simulink model "Gyrometer_model"  (R2015a)
settings: Solver=ode45  StartTime=0.0  StopTime=10.0  RelTol=1e-3
InitFcn:
  | Gyrometer_config;
undefined symbols (not defined in the file or in its folder): gyrometer
libraries: simulink x1
settings Model: Creator=hamada  LastModifiedBy=hamada

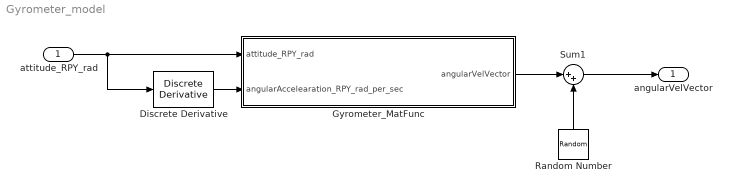
== system Gyrometer_model ==
  attitude_RPY_rad : Inport  PortDimensions=3
  Discrete Derivative : simulink/Discrete/Discrete Derivative  gainval=1.0  ICPrevScaledInput=0.0  InputProcessing=Inherited  OutMin=[]  OutMax=[]  OutDataType=fixdt(1, 16)  OutScaling=2^-10  DoSatur=off
  Gyrometer_MatFunc : MATLAB Function  TreatAsAtomicUnit=on
  Random Number : RandomNumber  Mean=gyrometer.bias  Variance=gyrometer.variance  SampleTime=gyrometer.period
  Sum1 : Sum  Inputs=|++
  angularVelVector : Outport
  wires:
  attitude_RPY_rad/1 -> Discrete Derivative/1, Gyrometer_MatFunc/1(attitude_RPY_rad)
  Gyrometer_MatFunc/1(angularVelVector) -> Sum1/1
  Random Number/1 -> Sum1/2
  Sum1/1 -> angularVelVector/1
  Discrete Derivative/1 -> Gyrometer_MatFunc/2(angularAccelearation_RPY_rad_per_sec)

== matlab function Gyrometer_model/Gyrometer_MatFunc ==
  data: attitude_RPY_rad input; angularAccelearation_RPY_rad_per_sec input; angularVelVector output
function angularVelVector = Gyrometer_MatFunc( attitude_RPY_rad, angularAccelearation_RPY_rad_per_sec )
    %#codegen
    angularVelVector = Gyrometer( attitude_RPY_rad, angularAccelearation_RPY_rad_per_sec  );
end
